simulink model "Step_20"  (R2024b)
settings: Solver=VariableStepAuto  StartTime=0.0  StopTime=10.0  RelTol=1e-3
libraries: simulink x1
settings Model: Creator=Omar

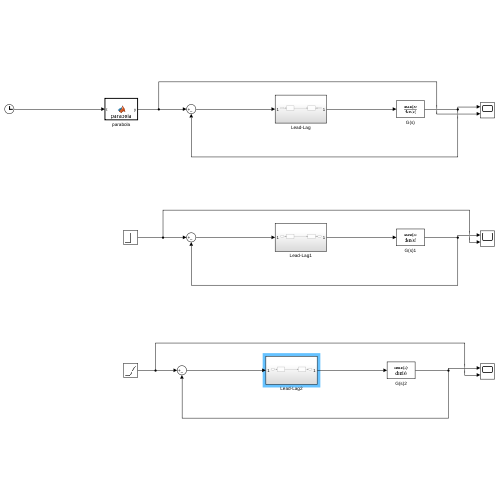
[thumbnail: Simulink's stored preview of the top-level diagram]
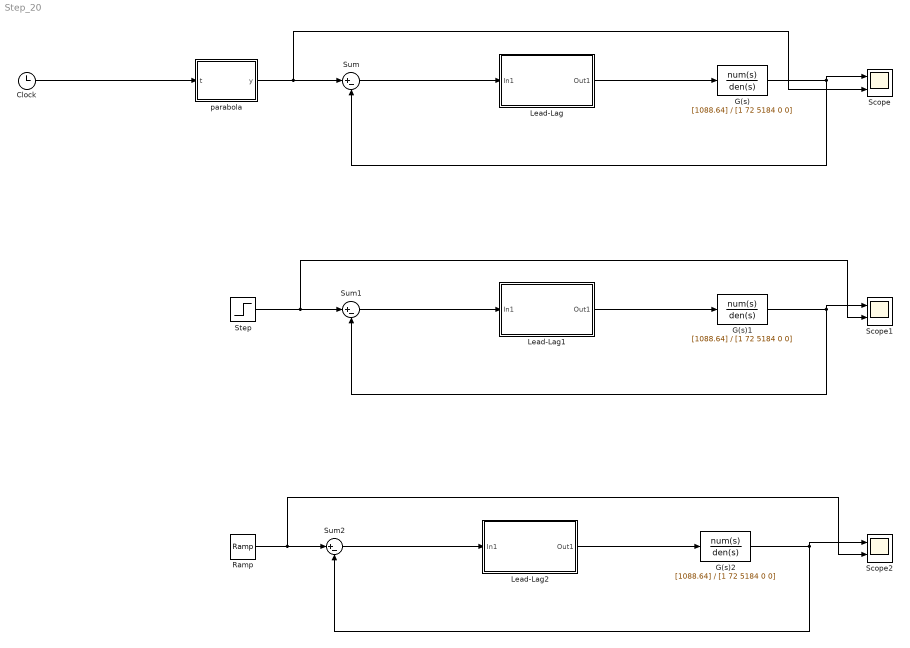
== system Step_20 ==
  Clock : Clock
      settings: Decimation=100
  G(s) : TransferFcn  Numerator=[1088.64]  Denominator=[1 72 5184 0 0]
  G(s)1 : TransferFcn  Numerator=[1088.64]  Denominator=[1 72 5184 0 0]
  G(s)2 : TransferFcn  Numerator=[1088.64]  Denominator=[1 72 5184 0 0]
  Lead-Lag : Subsystem
  Lead-Lag1 : Subsystem
  Lead-Lag2 : Subsystem
  Ramp : simulink/Sources/Ramp  slope=1  start=0  InitialOutput=0
  Scope : Scope  NumInputPorts=2
  Scope1 : Scope  NumInputPorts=2
  Scope2 : Scope  NumInputPorts=2
  Step : Step  SampleTime=0
  Sum : Sum  Inputs=|+-
  Sum1 : Sum  Inputs=|+-
  Sum2 : Sum  Inputs=|+-
  parabola : MATLAB Function  TreatAsAtomicUnit=on
  wires:
  Sum2/1 -> Lead-Lag2/1(In1)
  G(s)/1 -> Scope/1, Sum/2
  Sum1/1 -> Lead-Lag1/1(In1)
  parabola/1(y) -> Scope/2, Sum/1
  G(s)1/1 -> Scope1/1, Sum1/2
  Ramp/1 -> Scope2/2, Sum2/1
  Lead-Lag1/1(Out1) -> G(s)1/1
  Step/1 -> Scope1/2, Sum1/1
  G(s)2/1 -> Scope2/1, Sum2/2
  Sum/1 -> Lead-Lag/1(In1)
  Clock/1 -> parabola/1(t)
  Lead-Lag2/1(Out1) -> G(s)2/1
  Lead-Lag/1(Out1) -> G(s)/1

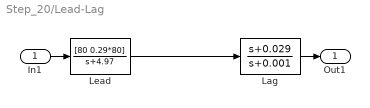
== system Step_20/Lead-Lag ==
  In1 : Inport
  Lag : TransferFcn  Numerator=[1 0.029]  Denominator=[1 0.001]
  Lead : TransferFcn  Numerator=[80 0.29*80]  Denominator=[1 4.97]
  Out1 : Outport
  wires:
  Lead/1 -> Lag/1
  Lag/1 -> Out1/1
  In1/1 -> Lead/1

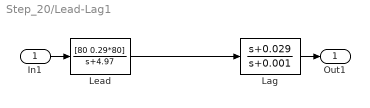
== system Step_20/Lead-Lag1 ==
  In1 : Inport
  Lag : TransferFcn  Numerator=[1 0.029]  Denominator=[1 0.001]
  Lead : TransferFcn  Numerator=[80 0.29*80]  Denominator=[1 4.97]
  Out1 : Outport
  wires:
  Lead/1 -> Lag/1
  Lag/1 -> Out1/1
  In1/1 -> Lead/1

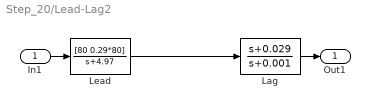
== system Step_20/Lead-Lag2 ==
  In1 : Inport
  Lag : TransferFcn  Numerator=[1 0.029]  Denominator=[1 0.001]
  Lead : TransferFcn  Numerator=[80 0.29*80]  Denominator=[1 4.97]
  Out1 : Outport
  wires:
  Lead/1 -> Lag/1
  Lag/1 -> Out1/1
  In1/1 -> Lead/1

== matlab function Step_20/parabola ==
  data: t input; y output
function y = parabola(t)
    a = 1; % Coefficient for t^2
    b = 0; % Coefficient for t
    c = 0; % Constant term
    y = a * t^2 + b * t + c;
end
